simulink model "tank_based_vv"  (R2020b)
settings: Solver=ode45  StartTime=0.0  StopTime=20  RelTol=1e-3
values from neighbouring files (symbols this model uses):
  alpha = 0.2    [hw7_main_vv.m]
  Amp = 0.8    [hw7_main_vv.m]
  Be = 20    [hw7_main_vv.m]
  beta = 0.2    [hw7_main_vv.m]
  Bh = 1.5    [hw7_main_vv.m]
  Bm = 1    [hw7_main_vv.m]
  Bs = 5    [hw7_main_vv.m]
  delay = 0    [hw7_main_vv.m]
  Dh = 8    [hw7_main_vv.m]
  Dm = 0    [hw7_main_vv.m]
  Ds = 0    [hw7_main_vv.m]
  Fc_lp = 5    [hw7_main_vv.m]
  Fc_sin = 0.1    [hw7_main_vv.m]
  H_D = 1    [hw7_main_vv.m]
  Je = 0    [hw7_main_vv.m]
  Jh = 0    [hw7_main_vv.m]
  Ke = 210    [hw7_main_vv.m]
  Kh = 0.1    [hw7_main_vv.m]
  Km = 5    [hw7_main_vv.m]
  Ks = 1    [hw7_main_vv.m]
  Mm = 0.5    [hw7_main_vv.m]
  Ms = 2    [hw7_main_vv.m]
  Ph = 1    [hw7_main_vv.m]
  Ts = 0.001    [hw7_main_vv.m]
  xe = 5    [hw7_main_vv.m]
libraries: simulink x2
settings Model: Creator=nicol  LastModifiedBy=nicol

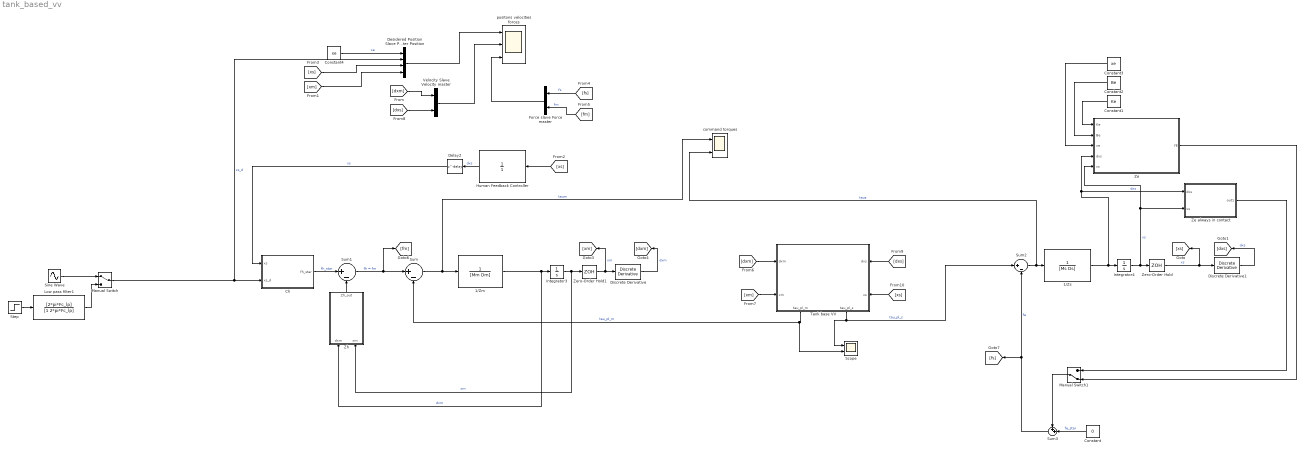
== system tank_based_vv ==
  1/Zm : TransferFcn  Denominator=[Mm Dm]
  1/Zs : TransferFcn  Denominator=[Ms Ds]
  Ch : Subsystem
  Constant : Constant  Value=0
  Constant1 : Constant  Value=Ke
  Constant2 : Constant  Value=Be
  Constant3 : Constant  Value=xe
  Constant4 : Constant  Value=xe
  Delay2 : Delay  DelayLength=delay  SampleTime=Ts
  Desidered Position Slave Position Master Position : Mux
  Discrete Derivative : simulink/Discrete/Discrete Derivative  gainval=1.0  ICPrevScaledInput=0.0  OutMin=[]  OutMax=[]  OutDataType=fixdt(1, 16)  OutScaling=2^-10  DoSatur=off
  Discrete Derivative1 : simulink/Discrete/Discrete Derivative  gainval=1.0  ICPrevScaledInput=0.0  OutMin=[]  OutMax=[]  OutDataType=fixdt(1, 16)  OutScaling=2^-10  DoSatur=off
  Force slave Force master : Mux  Inputs=2
  Human Feedback Controller : TransferFcn  Denominator=[1]
  Integrator3 : Integrator
  Integrator4 : Integrator
  Low pass filter1 : TransferFcn  Numerator=[2*pi*Fc_lp]  Denominator=[1 2*pi*Fc_lp]
  Manual Switch : ManualSwitch
  Manual Switch1 : ManualSwitch  CurrentSetting=0
  Scope : Scope  NumInputPorts=2
  Sine Wave : Sin  Amplitude=Amp  Frequency=2*pi*Fc_sin  SampleTime=0
  Step : Step  Time=Amp  After=Amp  SampleTime=0
  Sum : Sum  Inputs=|+-
  Sum1 : Sum  Inputs=|+-
  Sum2 : Sum  Inputs=|+-
  Sum3 : Sum  Inputs=++|
  Tank base VV : Subsystem
      settings: PortSchema="{\"entries\":[{\"content\":{\"sides\":[{\"content\":{\"connectorIds\":[\"In1\",\"In2\"]},\"type\":\"ConnectorPlacement.EquallySpacedRectSide\",\"uuid\":\"3a964002-fb37-4a92-b745-35f358b8e187\"},{\"content\":{\"connectorIds\":[\"In3\",\"In4\"],\"side\":\"RIGHT\"},\"type\":\"ConnectorPlacement.EquallySpacedRectSide\",\"uuid\":\"6a0ade08-0aa0-46a3-9e09-c310668c505c\"},{\"content\":{\"connectorIds\":[],\"side\":\"TOP\"},\"type\":\"ConnectorPlacement.EquallySpacedRectSide\",\"uuid\":\"1dfd7bbc-8185-4b5f-95de-42c58388ee02\"},{\"content\":{\"connectorIds\":[\"Out1\",\"Out2\"],\"side\":\"BOTTOM\"},\"type\":\"ConnectorPlacement.EquallySpacedRectSide\",\"uuid\":\"8c57ed43-4006-4572-ac50-c9adf88e8601\"},{\"content\":{\"connectorIds\":[],\"side\":\"HIDDEN\"},\"type\":\"ConnectorPlacement.EquallySpacedRectSide\",\"uuid\":\"15175a08-ca5b-4167-ba1d-f2e8cd3d814b\"}]},\"type\":\"ConnectorPlacement.EquallySpacedConnector\",\"uuid\":\"2bd1e993-3bc7-4875-9b20-3fb59092d5ec\"}],\"packageUris\":[\"http://schema.mathworks.com/mf0/Connector/R2020b\"],\"version\":\"1.0\"}"
  Velocity Slave Velocity master : Mux  Inputs=2
  Ze : MATLAB Function  TreatAsAtomicUnit=on
  Ze always in contact : Subsystem
  Zero-Order Hold : ZeroOrderHold  SampleTime=Ts
  Zero-Order Hold1 : ZeroOrderHold  SampleTime=Ts
  Zh : Subsystem
  command torques : Scope  NumInputPorts=2
  "positons velocities forces " : Scope  NumInputPorts=3
  wires:
  Ch/1(fh_star) -> Sum1/1  "fh_star"
  Zh/1(Zh_out) -> Sum1/2
  1/Zm/1 -> Zh/1(dxm), Integrator3/1  "dxm"
  Sum1/1 -> Sum/1, [fm]  "fh = fm"
  1/Zs/1 -> Integrator4/1, Ze always in contact/1(dxs), Ze/4(dxs)  "dxs"
  Sum2/1 -> 1/Zs/1, command torques/2  "taus"
  Ze/1(fE) -> Manual Switch1/2
  Sum3/1 -> [fs], Sum2/2  "fe"
  Constant/1 -> Sum3/2  "fe_star"
  Constant1/1 -> Ze/1(Ke)
  Constant2/1 -> Ze/2(Be)
  Constant3/1 -> Ze/3(xe)
  Integrator4/1 -> Zero-Order Hold/1, Ze/5(xs), Ze always in contact/2(xs)  "xs"
  Manual Switch1/1 -> Sum3/1
  Ze always in contact/1(out1) -> Manual Switch1/1
  Sum/1 -> command torques/1, 1/Zm/1  "taum"
  Velocity Slave Velocity master/1 -> "positons velocities forces "/2
  Desidered Position Slave Position Master Position/1 -> "positons velocities forces "/1
  Manual Switch/1 -> Desidered Position Slave Position Master Position/2, Ch/2(xs_d)  "xs_d"
  Discrete Derivative/1 -> [dxm]  "dxm"
  Zero-Order Hold1/1 -> [xm], Discrete Derivative/1  "xm"
  Integrator3/1 -> Zero-Order Hold1/1, Zh/2(xm)  "xm"
  Discrete Derivative1/1 -> [dxs]  "dxs"
  Zero-Order Hold/1 -> [xs], Discrete Derivative1/1  "xs"
  [xs] -> Human Feedback Controller/1
  Delay2/1 -> Ch/1(xs)  "xs"
  Human Feedback Controller/1 -> Delay2/1  "dxs"
  Sine Wave/1 -> Manual Switch/1
  [dxm] -> Velocity Slave Velocity master/1
  [xm] -> Desidered Position Slave Position Master Position/4
  [xs] -> Desidered Position Slave Position Master Position/3
  Constant4/1 -> Desidered Position Slave Position Master Position/1  "xe"
  Step/1 -> Low pass filter1/1
  [dxs] -> Velocity Slave Velocity master/2
  Low pass filter1/1 -> Manual Switch/2
  Force slave Force master/1 -> "positons velocities forces "/3
  [fs] -> Force slave Force master/1  "fs"
  [fm] -> Force slave Force master/2  "fm"
  [dxm] -> Tank base VV/1(dxm)
  [xm] -> Tank base VV/2(xm)
  [dxs] -> Tank base VV/3(dxs)
  [xs] -> Tank base VV/4(xs)
  Tank base VV/1(tau_pl_m) -> Scope/2, Sum/2  "tau_pl_m"
  Tank base VV/2(tau_pl_s) -> Sum2/1, Scope/1  "tau_pl_s"

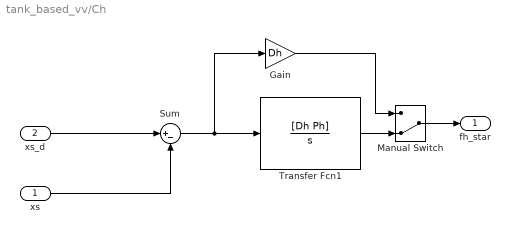
== system tank_based_vv/Ch ==
  xs : Inport
  xs_d : Inport  Port=2
  Gain : Gain  Gain=Dh
  Manual Switch : ManualSwitch  CurrentSetting=0
  Sum : Sum  Inputs=|+-
  Transfer Fcn1 : TransferFcn  Numerator=[Dh Ph]  Denominator=[1 0]
  fh_star : Outport
  wires:
  xs/1 -> Sum/2
  Sum/1 -> Gain/1, Transfer Fcn1/1
  Transfer Fcn1/1 -> Manual Switch/2
  xs_d/1 -> Sum/1
  Manual Switch/1 -> fh_star/1
  Gain/1 -> Manual Switch/1

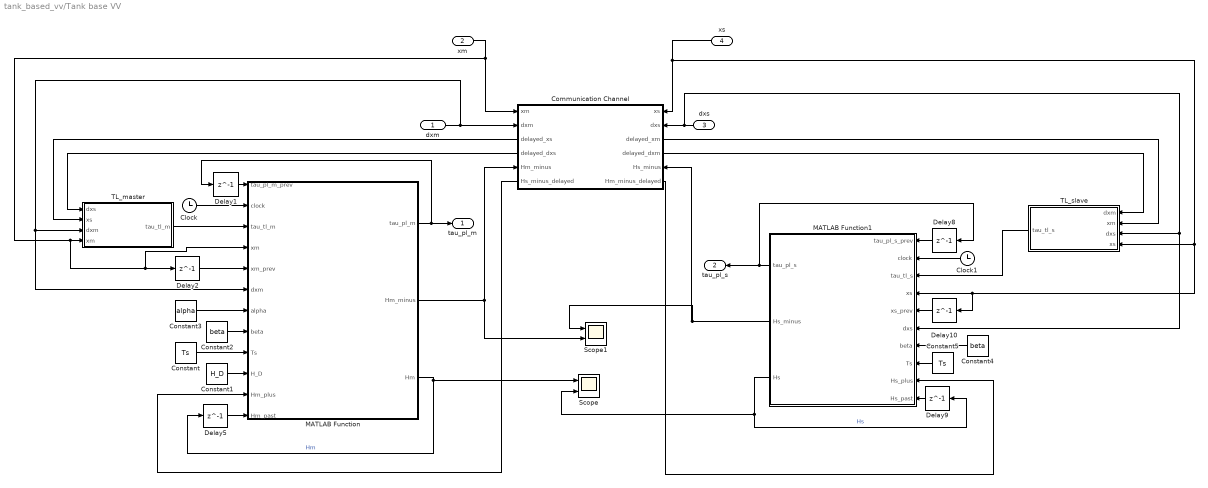
== system tank_based_vv/Tank base VV ==
  dxm : Inport
  xm : Inport  Port=2
  dxs : Inport  Port=3
  xs : Inport  Port=4
  Clock : Clock
  Clock1 : Clock
  Communication Channel : Subsystem
      settings: PortSchema="{\"entries\":[{\"content\":{\"sides\":[{\"content\":{\"connectorIds\":[\"In1\",\"In2\",\"Out4\",\"Out5\",\"In3\",\"Out6\"]},\"type\":\"ConnectorPlacement.EquallySpacedRectSide\",\"uuid\":\"707b854d-ad7a-498f-bed1-9a4f8657ce88\"},{\"content\":{\"connectorIds\":[\"In4\",\"In5\",\"Out1\",\"Out2\",\"In6\",\"Out3\"],\"side\":\"RIGHT\"},\"type\":\"ConnectorPlacement.EquallySpacedRectSide\",\"uuid\":\"12f3e034-857d-4081-a3d0-204c7e32b1d7\"},{\"content\":{\"connectorIds\":[],\"side\":\"TOP\"},\"type\":\"ConnectorPlacement.EquallySpacedRectSide\",\"uuid\":\"fb6b09f7-6084-4258-a6c2-180f375b33c2\"},{\"content\":{\"connectorIds\":[],\"side\":\"HIDDEN\"},\"type\":\"ConnectorPlacement.EquallySpacedRectSide\",\"uuid\":\"424096ec-dcd8-463d-bba6-855fd00452bd\"}]},\"type\":\"ConnectorPlacement.EquallySpacedConnector\",\"uuid\":\"13b09cb8-9f61-41a9-b654-31f5f7de73c5\"}],\"packageUris\":[\"http://schema.mathworks.com/mf0/Connector/R2020b\"],\"version\":\"1.0\"}"
  Constant : Constant  Value=Ts
  Constant1 : Constant  Value=H_D
  Constant2 : Constant  Value=beta
  Constant3 : Constant  Value=alpha
  Constant4 : Constant  Value=beta
  Constant5 : Constant  Value=Ts
  Delay{1..2,5,8..10} (6 alike) : Delay  DelayLength=1
  MATLAB Function : MATLAB Function  TreatAsAtomicUnit=on
  MATLAB Function1 : MATLAB Function  TreatAsAtomicUnit=on
  Scope : Scope  NumInputPorts=2
  Scope1 : Scope  NumInputPorts=2
  TL_master : Subsystem
  TL_slave : Subsystem
  tau_pl_m : Outport
  tau_pl_s : Outport  Port=2
  wires:
  TL_master/1(tau_tl_m) -> MATLAB Function/3(tau_tl_m)
  TL_slave/1(tau_tl_s) -> MATLAB Function1/3(tau_tl_s)
  Clock/1 -> MATLAB Function/2(clock)
  MATLAB Function/1(tau_pl_m) -> Delay1/1, tau_pl_m/1
  Delay1/1 -> MATLAB Function/1(tau_pl_m_prev)
  Delay2/1 -> MATLAB Function/5(xm_prev)
  Delay5/1 -> MATLAB Function/12(Hm_past)
  Constant/1 -> MATLAB Function/9(Ts)
  Constant1/1 -> MATLAB Function/10(H_D)
  MATLAB Function/3(Hm) -> Delay5/1, Scope/1  "Hm"
  Constant2/1 -> MATLAB Function/8(beta)
  Constant3/1 -> MATLAB Function/7(alpha)
  Communication Channel/3(Hs_minus_delayed) -> MATLAB Function/11(Hm_plus)
  MATLAB Function1/1(tau_pl_s) -> Delay8/1, tau_pl_s/1
  Delay8/1 -> MATLAB Function1/1(tau_pl_s_prev)
  Clock1/1 -> MATLAB Function1/2(clock)
  Constant4/1 -> MATLAB Function1/7(beta)
  Constant5/1 -> MATLAB Function1/8(Ts)
  Delay9/1 -> MATLAB Function1/10(Hs_past)
  MATLAB Function1/3(Hs) -> Scope/2, Delay9/1  "Hs"
  Delay10/1 -> MATLAB Function1/5(xs_prev)
  xs/1 -> Communication Channel/1(xs), Delay10/1, MATLAB Function1/4(xs), TL_slave/4(xs)
  xm/1 -> Communication Channel/4(xm), MATLAB Function/4(xm), Delay2/1, TL_master/4(xm)
  dxm/1 -> MATLAB Function/6(dxm), TL_master/3(dxm), Communication Channel/5(dxm)
  dxs/1 -> Communication Channel/2(dxs), MATLAB Function1/6(dxs), TL_slave/3(dxs)
  MATLAB Function/2(Hm_minus) -> Scope1/2, Communication Channel/6(Hm_minus)
  MATLAB Function1/2(Hs_minus) -> Scope1/1, Communication Channel/3(Hs_minus)
  Communication Channel/6(Hm_minus_delayed) -> MATLAB Function1/9(Hs_plus)
  Communication Channel/4(delayed_xm) -> TL_slave/2(xm)
  Communication Channel/5(delayed_dxm) -> TL_slave/1(dxm)
  Communication Channel/1(delayed_xs) -> TL_master/2(xs)
  Communication Channel/2(delayed_dxs) -> TL_master/1(dxs)

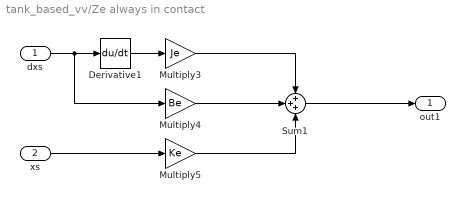
== system tank_based_vv/Ze always in contact ==
  dxs : Inport
  xs : Inport  Port=2
  Derivative1 : Derivative
  Multiply3 : Gain  Gain=Je
  Multiply4 : Gain  Gain=Be
  Multiply5 : Gain  Gain=Ke
  Sum1 : Sum  Inputs=+++
  out1 : Outport
  wires:
  Sum1/1 -> out1/1
  Multiply4/1 -> Sum1/2
  Multiply5/1 -> Sum1/3
  dxs/1 -> Multiply4/1, Derivative1/1
  Derivative1/1 -> Multiply3/1
  xs/1 -> Multiply5/1
  Multiply3/1 -> Sum1/1

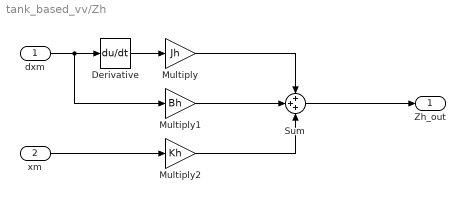
== system tank_based_vv/Zh ==
  dxm : Inport
  xm : Inport  Port=2
  Derivative : Derivative
  Multiply : Gain  Gain=Jh
  Multiply1 : Gain  Gain=Bh
  Multiply2 : Gain  Gain=Kh
  Sum : Sum  Inputs=+++
  Zh_out : Outport
  wires:
  dxm/1 -> Multiply1/1, Derivative/1
  Derivative/1 -> Multiply/1
  Sum/1 -> Zh_out/1
  xm/1 -> Multiply2/1
  Multiply1/1 -> Sum/2
  Multiply/1 -> Sum/1
  Multiply2/1 -> Sum/3

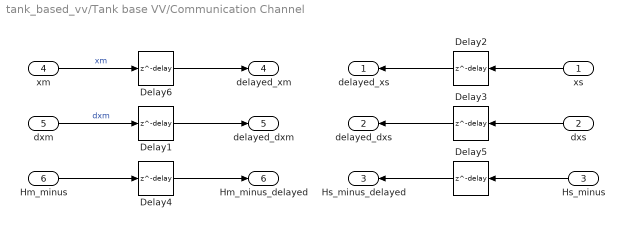
== system tank_based_vv/Tank base VV/Communication Channel ==
  xs : Inport
  dxs : Inport  Port=2
  Hs_minus : Inport  Port=3
  xm : Inport  Port=4
  dxm : Inport  Port=5
  Hm_minus : Inport  Port=6
  Delay{1..6} (6 alike) : Delay  DelayLength=delay  SampleTime=Ts
  delayed_xs : Outport
  delayed_dxs : Outport  Port=2
  Hs_minus_delayed : Outport  Port=3
  delayed_xm : Outport  Port=4
  delayed_dxm : Outport  Port=5
  Hm_minus_delayed : Outport  Port=6
  wires:
  xm/1 -> Delay6/1  "xm"
  dxm/1 -> Delay1/1  "dxm"
  Delay6/1 -> delayed_xm/1
  Delay1/1 -> delayed_dxm/1
  Delay3/1 -> delayed_dxs/1
  xs/1 -> Delay2/1
  dxs/1 -> Delay3/1
  Delay2/1 -> delayed_xs/1
  Hm_minus/1 -> Delay4/1
  Delay4/1 -> Hm_minus_delayed/1
  Delay5/1 -> Hs_minus_delayed/1
  Hs_minus/1 -> Delay5/1

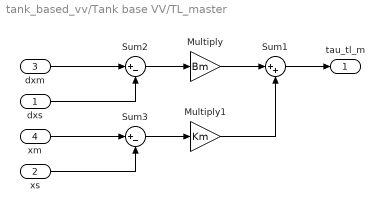
== system tank_based_vv/Tank base VV/TL_master ==
  dxs : Inport
  xs : Inport  Port=2
  dxm : Inport  Port=3
  xm : Inport  Port=4
  Multiply : Gain  Gain=Bm
  Multiply1 : Gain  Gain=Km
  Sum1 : Sum  Inputs=|++
  Sum2 : Sum  Inputs=|+-
  Sum3 : Sum  Inputs=|+-
  tau_tl_m : Outport
  wires:
  Sum2/1 -> Multiply/1
  Multiply1/1 -> Sum1/2
  Multiply/1 -> Sum1/1
  Sum1/1 -> tau_tl_m/1
  Sum3/1 -> Multiply1/1
  xm/1 -> Sum3/1
  xs/1 -> Sum3/2
  dxs/1 -> Sum2/2
  dxm/1 -> Sum2/1

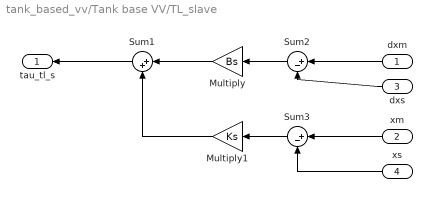
== system tank_based_vv/Tank base VV/TL_slave ==
  dxm : Inport
  xm : Inport  Port=2
  dxs : Inport  Port=3
  xs : Inport  Port=4
  Multiply : Gain  Gain=Bs
  Multiply1 : Gain  Gain=Ks
  Sum1 : Sum  Inputs=|++
  Sum2 : Sum  Inputs=|+-
  Sum3 : Sum  Inputs=|+-
  tau_tl_s : Outport
  wires:
  Sum2/1 -> Multiply/1
  Multiply1/1 -> Sum1/2
  Multiply/1 -> Sum1/1
  Sum1/1 -> tau_tl_s/1
  Sum3/1 -> Multiply1/1
  xm/1 -> Sum3/1
  xs/1 -> Sum3/2
  dxs/1 -> Sum2/2
  dxm/1 -> Sum2/1

== matlab function tank_based_vv/Tank base VV/MATLAB Function ==
  data: tau_pl_m_prev input; clock input; tau_pl_m output; Hm_minus output; tau_tl_m input; xm input; xm_prev input; dxm input; alpha input; beta input; Ts input; H_D input; Hm_plus input; Hm_past input; Hm output
function [tau_pl_m, Hm_minus, Hm] = passivity_layer_master(tau_pl_m_prev, clock, tau_tl_m, xm, xm_prev, dxm, alpha, beta, Ts, H_D, Hm_plus, Hm_past)
    if clock == 0
        Hm_past = 0;
        tau_pl_m_prev = 0; 
    end
    
    delta_xm = xm - xm_prev;
    delta_H_used = tau_pl_m_prev*(delta_xm);
    H = Hm_past + Hm_plus - delta_H_used;

    % Compute tau limits
    if H <= 0 
        tau_max_m_1 = 0;
    else
        tau_max_m_1 = tau_tl_m;
    end
    
    if abs(dxm) < 0.001
        tau_max_m_2 = sign(dxm)*1e9;
    else
        tau_max_m_2 =  H/(dxm*Ts);
    end
    
    tau_pl_m_sup = sign(tau_tl_m)*min(abs(tau_max_m_1), abs(tau_max_m_2));

    % TLC check
    if(H < H_D)
       d = alpha*(H_D - H);
       tau_TLC = -d*dxm;
       tau_pl_m = tau_pl_m_sup + tau_TLC;
    else
        tau_pl_m = tau_pl_m_sup;
    end
    
    % Send energy
    Hm_minus = 0;
    if (H > 0)
        Hm_minus =  beta*H;
        Hm = H - Hm_minus;  
    else
        Hm = 0;
    end
end

== matlab function tank_based_vv/Ze ==
  data: Ke input; fE output; Be input; xe input; dxs input; xs input
function fE = environment(Ke, Be, xe, dxs, xs)
if(xs > xe)
    fE = Ke*(xs - xe) + Be*dxs;
else
    fE=0;
end

== matlab function tank_based_vv/Tank base VV/MATLAB Function1 ==
  data: tau_pl_s output; Hs_minus output; tau_pl_s_prev input; Hs output; clock input; tau_tl_s input; xs input; xs_prev input; dxs input; beta input; Ts input; Hs_plus input; Hs_past input
function [tau_pl_s, Hs_minus, Hs] = passivity_master_slave(tau_pl_s_prev, clock, tau_tl_s, xs, xs_prev, dxs, beta, Ts, Hs_plus, Hs_past)
    if clock == 0
        Hs_past = 0;
        tau_pl_s_prev = 0; 
    end
    
    delta_xs = xs - xs_prev;
    delta_H_used = tau_pl_s_prev*(delta_xs);
    H = Hs_past + Hs_plus - delta_H_used;

    % Compute tau limits
    if H <= 0 
        tau_max_s_1 = 0;
    else
        tau_max_s_1 = tau_tl_s;
    end
    
    if abs(dxs) < 0.001
        tau_max_s_2 = sign(dxs)*1e9;
    else
        tau_max_s_2 =  H/(dxs*Ts);
    end
    
    tau_pl_s = sign(tau_tl_s)*min(abs(tau_max_s_1), abs(tau_max_s_2));
    
    % Send energy
    Hs_minus = 0;
    if (H > 0)
        Hs_minus =  beta*H;
        Hs = H - Hs_minus;  
    else
        Hs = 0;
    end
end
